simulink model "KTB1_EKF2b"  (R2022b)
settings: Solver=ode23tb  StartTime=0.0  StopTime=500  RelTol=1e-3
libraries: slpidlib x6
settings Model: Creator=s182032  LastModifiedBy=morebo
settings DataIOCC: ReturnWorkspaceOutputs=off
settings DebuggingCC: MaxConsecutiveZCsMsg=none  UnconnectedInputMsg=warning  UnconnectedOutputMsg=warning  UnconnectedLineMsg=warning  SFMachineParentedDataDiag=warning  ArithmeticOperatorsInVariantConditions=warning
settings ModelReferenceCC: EnableRefExpFcnMdlSchedulingChecks=on
settings SFSimCC: SimUseLocalCustomCode=off  CustomCodeUndefinedFunction=UseInterfaceOnly
settings RTWCC: RTWUseLocalCustomCode=off

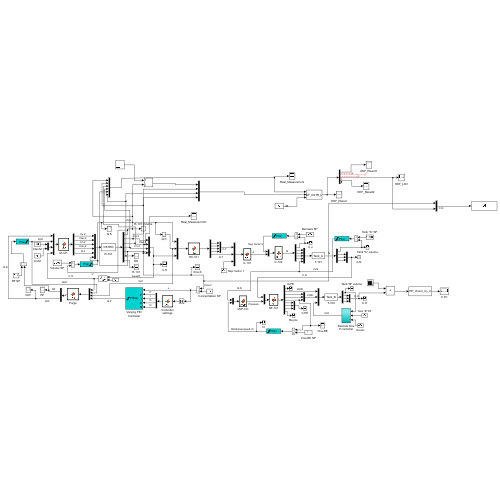
[thumbnail: Simulink's stored preview of the top-level diagram]
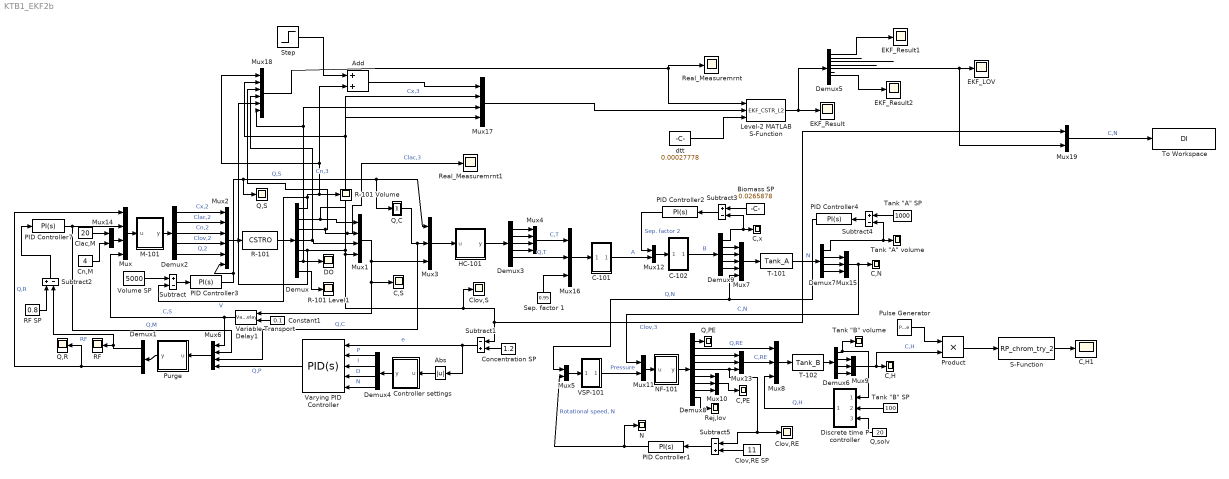
== system KTB1_EKF2b ==
  Abs : Abs  SaturateOnIntegerOverflow=off
  Add : Sum
  Biomass SP : Constant  Value=0.0265878
  C,H : Scope
  C,H1 : Scope
  C,N : Scope
  C,PE : Scope
  C,S : Scope
  C,x : Scope
  C-101 : MATLAB Function  TreatAsAtomicUnit=on
  C-102 : MATLAB Function  TreatAsAtomicUnit=on
  Clac,M : Constant  Value=20
  Clov,RE : Scope
  Clov,RE SP : Constant  Value=11
  Clov,S : Scope
  Cn,M : Constant  Value=4
  Concentration SP : Constant  Value=1.2
  Constant1 : Constant  Value=0.1
  Controller settings : MATLAB Function  TreatAsAtomicUnit=on
  DO : Scope
  Demux : Demux  Outputs=7
  Demux1 : Demux  Outputs=2
  Demux2 : Demux  Outputs=5
  Demux3 : Demux  Outputs=5
  Demux4 : Demux
  Demux5 : Demux  Outputs=8
  Demux6 : Demux
  Demux7 : Demux
  Demux8 : Demux  Outputs=9
  Demux9 : Demux  Outputs=5
  Discrete time P controller : Subsystem
  EKF_LOV : Scope
  EKF_Result : Scope
  EKF_Result1 : Scope
  EKF_Result2 : Scope
  HC-101 : MATLAB Function  TreatAsAtomicUnit=on
  Level-2 MATLAB S-Function : M-S-Function  FunctionName=EKF_CSTR_L2
  M-101 : MATLAB Function  TreatAsAtomicUnit=on
  Mux{,1,4,6,17} (5 alike) : Mux
  Mux{3,8..10,13,15..16} (7 alike) : Mux  Inputs=3
  Mux{5,11..12,14,19} (5 alike) : Mux  Inputs=2
  Mux18 : Mux  Inputs=6
  Mux2 : Mux  Inputs=6
  Mux7 : Mux  Inputs=5
  N : Scope
  NF-101 : MATLAB Function  TreatAsAtomicUnit=on
  PID Controller1 : slpidlib/PID Controller  Controller=PI  Form=Parallel  TimeDomain=Continuous-time  UseExternalTs=off  SampleTime=-1  IntegratorMethod=Forward Euler  FilterMethod=Forward Euler  ControllerParametersSource=internal  P=0.234567821807165  I=0.999999996666666*0.234567821807165  UseKiTs=off  D=0  N=100  UseFilter=on  TunerSelectOption=Transfer Function Based (PID Tuner App)  InitialConditionSource=internal  InitialConditionForIntegrator=3000  InitialConditionForFilter=0  DifferentiatorICPrevScaledInput=0  ExternalReset=none  TrackingMode=off  Kt=1  LimitOutput=on  SatLimitsSource=internal  UpperSaturationLimit=inf  LowerSaturationLimit=0  LinearizeAsGain=on  AntiWindupMode=clamping  Kb=1  LimitIntegrator=off  UpperIntegratorSaturationLimit=inf  LowerIntegratorSaturationLimit=-inf  POutMin=[]  POutMax=[]  IOutMin=[]  IOutMax=[]  DOutMin=[]  DOutMax=[]  NOutMin=[]  NOutMax=[]  SumOutMin=[]  SumOutMax=[]  SaturationOutMin=[]  SaturationOutMax=[]  PParamMin=[]  PParamMax=[]  IParamMin=[]  IParamMax=[]  DParamMin=[]  DParamMax=[]  NParamMin=[]  NParamMax=[]  KbParamMin=[]  KbParamMax=[]  KtParamMin=[]  KtParamMax=[]  KbOutMin=[]  KbOutMax=[]  KtOutMin=[]  KtOutMax=[]  IntegratorOutMin=[]  IntegratorOutMax=[]  FilterOutMin=[]  FilterOutMax=[]  SumI1OutMin=[]  SumI1OutMax=[]  SumI2OutMin=[]  SumI2OutMax=[]  SumI3OutMin=[]  SumI3OutMax=[]  SumI4OutMin=[]  SumI4OutMax=[]  SumDOutMin=[]  SumDOutMax=[]  DifferentiatorOutMin=[]  DifferentiatorOutMax=[]  FilterDiffOutCoefMin=[]  FilterDiffOutCoefMax=[]  ReciprocalOutMin=[]  ReciprocalOutMax=[]  SumDenOutMin=[]  SumDenOutMax=[]  SumNumOutMin=[]  SumNumOutMax=[]  DivideOutMin=[]  DivideOutMax=[]  UdiffTsProdOutMin=[]  UdiffTsProdOutMax=[]  NTsProdOutMin=[]  NTsProdOutMax=[]  UintegralTsProdOutMin=[]  UintegralTsProdOutMax=[]  UngainTsProdOutMin=[]  UngainTsProdOutMax=[]  ClampingZeroOutDataTypeStr=Inherit: Inherit via back propagation  ClampingZeroOutMin=[]  ClampingZeroOutMax=[]  FilterDenConstantOutDataTypeStr=Inherit: Inherit via back propagation  FilterDenConstantOutMin=[]  FilterDenConstantOutMax=[]  PCopyOutDataTypeStr=Inherit: Inherit via back propagation  PCopyOutMin=[]  PCopyOutMax=[]  NCopyOutDataTypeStr=Inherit: Inherit via back propagation  NCopyOutMin=[]  NCopyOutMax=[]  IntegratorContinuousStateAttributes=''  IntegratorStateMustResolveToSignalObject=off  IntegratorRTWStateStorageClass=Auto  FilterContinuousStateAttributes=''  FilterStateMustResolveToSignalObject=off  FilterRTWStateStorageClass=Auto  ParallelPVariant=InternalParameters  IdealPVariant=Disabled  IVariant=InternalParameters  DVariant=Disabled  IntegratorVariant=Continuous  SatVariant=Enabled  AWVariant=ContClampingParallel  PCopyVariant=Disabled  TRVariant=Disabled  FdbkBlocksVariant=Forward  IdealPFdbkVariant=Disabled  SatFdbkVariant=Disabled  DerivativeFilterVariant=Disabled  NVariant=Disabled  NCopyVariant=Disabled_SignalSpec  FilterICVariant=Disabled  IntegratorICVariant=InternalICs  ExternalResetVariant=Disabled  TRSumVariant=Passthrough  SumFdbkVariant=Disabled  SumVariant=Sum_PI  TsampFilterVariant=InternalTs  TsampNgainVariant=Passthrough  TsampIntegralVariant=Passthrough  ExternalSaturationOutDataTypeStr=Inherit: Same as second input
  PID Controller2 : slpidlib/PID Controller  Controller=PI  Form=Parallel  TimeDomain=Continuous-time  UseExternalTs=off  SampleTime=-1  IntegratorMethod=Forward Euler  FilterMethod=Forward Euler  ControllerParametersSource=internal  P=-0.000476190628986061  I=9.99999996666667*(-0.000476190628986061)  UseKiTs=off  D=0  N=100  UseFilter=on  TunerSelectOption=Transfer Function Based (PID Tuner App)  InitialConditionSource=internal  InitialConditionForIntegrator=0.95  InitialConditionForFilter=0  DifferentiatorICPrevScaledInput=0  ExternalReset=none  TrackingMode=off  Kt=1  LimitOutput=on  SatLimitsSource=internal  UpperSaturationLimit=0.98  LowerSaturationLimit=0  LinearizeAsGain=on  AntiWindupMode=clamping  Kb=1  LimitIntegrator=off  UpperIntegratorSaturationLimit=inf  LowerIntegratorSaturationLimit=-inf  POutMin=[]  POutMax=[]  IOutMin=[]  IOutMax=[]  DOutMin=[]  DOutMax=[]  NOutMin=[]  NOutMax=[]  SumOutMin=[]  SumOutMax=[]  SaturationOutMin=[]  SaturationOutMax=[]  PParamMin=[]  PParamMax=[]  IParamMin=[]  IParamMax=[]  DParamMin=[]  DParamMax=[]  NParamMin=[]  NParamMax=[]  KbParamMin=[]  KbParamMax=[]  KtParamMin=[]  KtParamMax=[]  KbOutMin=[]  KbOutMax=[]  KtOutMin=[]  KtOutMax=[]  IntegratorOutMin=[]  IntegratorOutMax=[]  FilterOutMin=[]  FilterOutMax=[]  SumI1OutMin=[]  SumI1OutMax=[]  SumI2OutMin=[]  SumI2OutMax=[]  SumI3OutMin=[]  SumI3OutMax=[]  SumI4OutMin=[]  SumI4OutMax=[]  SumDOutMin=[]  SumDOutMax=[]  DifferentiatorOutMin=[]  DifferentiatorOutMax=[]  FilterDiffOutCoefMin=[]  FilterDiffOutCoefMax=[]  ReciprocalOutMin=[]  ReciprocalOutMax=[]  SumDenOutMin=[]  SumDenOutMax=[]  SumNumOutMin=[]  SumNumOutMax=[]  DivideOutMin=[]  DivideOutMax=[]  UdiffTsProdOutMin=[]  UdiffTsProdOutMax=[]  NTsProdOutMin=[]  NTsProdOutMax=[]  UintegralTsProdOutMin=[]  UintegralTsProdOutMax=[]  UngainTsProdOutMin=[]  UngainTsProdOutMax=[]  ClampingZeroOutDataTypeStr=Inherit: Inherit via back propagation  ClampingZeroOutMin=[]  ClampingZeroOutMax=[]  FilterDenConstantOutDataTypeStr=Inherit: Inherit via back propagation  FilterDenConstantOutMin=[]  FilterDenConstantOutMax=[]  PCopyOutDataTypeStr=Inherit: Inherit via back propagation  PCopyOutMin=[]  PCopyOutMax=[]  NCopyOutDataTypeStr=Inherit: Inherit via back propagation  NCopyOutMin=[]  NCopyOutMax=[]  IntegratorContinuousStateAttributes=''  IntegratorStateMustResolveToSignalObject=off  IntegratorRTWStateStorageClass=Auto  FilterContinuousStateAttributes=''  FilterStateMustResolveToSignalObject=off  FilterRTWStateStorageClass=Auto  ParallelPVariant=InternalParameters  IdealPVariant=Disabled  IVariant=InternalParameters  DVariant=Disabled  IntegratorVariant=Continuous  SatVariant=Enabled  AWVariant=ContClampingParallel  PCopyVariant=Disabled  TRVariant=Disabled  FdbkBlocksVariant=Forward  IdealPFdbkVariant=Disabled  SatFdbkVariant=Disabled  DerivativeFilterVariant=Disabled  NVariant=Disabled  NCopyVariant=Disabled_SignalSpec  FilterICVariant=Disabled  IntegratorICVariant=InternalICs  ExternalResetVariant=Disabled  TRSumVariant=Passthrough  SumFdbkVariant=Disabled  SumVariant=Sum_PI  TsampFilterVariant=InternalTs  TsampNgainVariant=Passthrough  TsampIntegralVariant=Passthrough  ExternalSaturationOutDataTypeStr=Inherit: Same as second input
  PID Controller3 : slpidlib/PID Controller  Controller=PI  Form=Parallel  TimeDomain=Continuous-time  UseExternalTs=off  SampleTime=-1  IntegratorMethod=Forward Euler  FilterMethod=Forward Euler  ControllerParametersSource=internal  P=-1/0.4/0.2  I=-1/0.4/0.2/4/0.2  UseKiTs=off  D=0  N=100  UseFilter=on  TunerSelectOption=Transfer Function Based (PID Tuner App)  InitialConditionSource=internal  InitialConditionForIntegrator=64.0830509473650  InitialConditionForFilter=0  DifferentiatorICPrevScaledInput=0  ExternalReset=none  TrackingMode=off  Kt=1  LimitOutput=on  SatLimitsSource=internal  UpperSaturationLimit=inf  LowerSaturationLimit=0  LinearizeAsGain=on  AntiWindupMode=clamping  Kb=1  LimitIntegrator=off  UpperIntegratorSaturationLimit=inf  LowerIntegratorSaturationLimit=-inf  POutMin=[]  POutMax=[]  IOutMin=[]  IOutMax=[]  DOutMin=[]  DOutMax=[]  NOutMin=[]  NOutMax=[]  SumOutMin=[]  SumOutMax=[]  SaturationOutMin=[]  SaturationOutMax=[]  PParamMin=[]  PParamMax=[]  IParamMin=[]  IParamMax=[]  DParamMin=[]  DParamMax=[]  NParamMin=[]  NParamMax=[]  KbParamMin=[]  KbParamMax=[]  KtParamMin=[]  KtParamMax=[]  KbOutMin=[]  KbOutMax=[]  KtOutMin=[]  KtOutMax=[]  IntegratorOutMin=[]  IntegratorOutMax=[]  FilterOutMin=[]  FilterOutMax=[]  SumI1OutMin=[]  SumI1OutMax=[]  SumI2OutMin=[]  SumI2OutMax=[]  SumI3OutMin=[]  SumI3OutMax=[]  SumI4OutMin=[]  SumI4OutMax=[]  SumDOutMin=[]  SumDOutMax=[]  DifferentiatorOutMin=[]  DifferentiatorOutMax=[]  FilterDiffOutCoefMin=[]  FilterDiffOutCoefMax=[]  ReciprocalOutMin=[]  ReciprocalOutMax=[]  SumDenOutMin=[]  SumDenOutMax=[]  SumNumOutMin=[]  SumNumOutMax=[]  DivideOutMin=[]  DivideOutMax=[]  UdiffTsProdOutMin=[]  UdiffTsProdOutMax=[]  NTsProdOutMin=[]  NTsProdOutMax=[]  UintegralTsProdOutMin=[]  UintegralTsProdOutMax=[]  UngainTsProdOutMin=[]  UngainTsProdOutMax=[]  ClampingZeroOutDataTypeStr=Inherit: Inherit via back propagation  ClampingZeroOutMin=[]  ClampingZeroOutMax=[]  FilterDenConstantOutDataTypeStr=Inherit: Inherit via back propagation  FilterDenConstantOutMin=[]  FilterDenConstantOutMax=[]  PCopyOutDataTypeStr=Inherit: Inherit via back propagation  PCopyOutMin=[]  PCopyOutMax=[]  NCopyOutDataTypeStr=Inherit: Inherit via back propagation  NCopyOutMin=[]  NCopyOutMax=[]  IntegratorContinuousStateAttributes=''  IntegratorStateMustResolveToSignalObject=off  IntegratorRTWStateStorageClass=Auto  FilterContinuousStateAttributes=''  FilterStateMustResolveToSignalObject=off  FilterRTWStateStorageClass=Auto  ParallelPVariant=InternalParameters  IdealPVariant=Disabled  IVariant=InternalParameters  DVariant=Disabled  IntegratorVariant=Continuous  SatVariant=Enabled  AWVariant=ContClampingParallel  PCopyVariant=Disabled  TRVariant=Disabled  FdbkBlocksVariant=Forward  IdealPFdbkVariant=Disabled  SatFdbkVariant=Disabled  DerivativeFilterVariant=Disabled  NVariant=Disabled  NCopyVariant=Disabled_SignalSpec  FilterICVariant=Disabled  IntegratorICVariant=InternalICs  ExternalResetVariant=Disabled  TRSumVariant=Passthrough  SumFdbkVariant=Disabled  SumVariant=Sum_PI  TsampFilterVariant=InternalTs  TsampNgainVariant=Passthrough  TsampIntegralVariant=Passthrough  ExternalSaturationOutDataTypeStr=Inherit: Same as second input
  PID Controller4 : slpidlib/PID Controller  Controller=PI  Form=Parallel  TimeDomain=Continuous-time  UseExternalTs=off  SampleTime=-1  IntegratorMethod=Forward Euler  FilterMethod=Forward Euler  ControllerParametersSource=internal  P=-1/140  I=-1/4/140/140  UseKiTs=off  D=0  N=100  UseFilter=on  TunerSelectOption=Transfer Function Based (PID Tuner App)  InitialConditionSource=internal  InitialConditionForIntegrator=25.6332203789471  InitialConditionForFilter=0  DifferentiatorICPrevScaledInput=0  ExternalReset=none  TrackingMode=off  Kt=1  LimitOutput=on  SatLimitsSource=internal  UpperSaturationLimit=inf  LowerSaturationLimit=0  LinearizeAsGain=on  AntiWindupMode=clamping  Kb=1  LimitIntegrator=off  UpperIntegratorSaturationLimit=inf  LowerIntegratorSaturationLimit=-inf  POutMin=[]  POutMax=[]  IOutMin=[]  IOutMax=[]  DOutMin=[]  DOutMax=[]  NOutMin=[]  NOutMax=[]  SumOutMin=[]  SumOutMax=[]  SaturationOutMin=[]  SaturationOutMax=[]  PParamMin=[]  PParamMax=[]  IParamMin=[]  IParamMax=[]  DParamMin=[]  DParamMax=[]  NParamMin=[]  NParamMax=[]  KbParamMin=[]  KbParamMax=[]  KtParamMin=[]  KtParamMax=[]  KbOutMin=[]  KbOutMax=[]  KtOutMin=[]  KtOutMax=[]  IntegratorOutMin=[]  IntegratorOutMax=[]  FilterOutMin=[]  FilterOutMax=[]  SumI1OutMin=[]  SumI1OutMax=[]  SumI2OutMin=[]  SumI2OutMax=[]  SumI3OutMin=[]  SumI3OutMax=[]  SumI4OutMin=[]  SumI4OutMax=[]  SumDOutMin=[]  SumDOutMax=[]  DifferentiatorOutMin=[]  DifferentiatorOutMax=[]  FilterDiffOutCoefMin=[]  FilterDiffOutCoefMax=[]  ReciprocalOutMin=[]  ReciprocalOutMax=[]  SumDenOutMin=[]  SumDenOutMax=[]  SumNumOutMin=[]  SumNumOutMax=[]  DivideOutMin=[]  DivideOutMax=[]  UdiffTsProdOutMin=[]  UdiffTsProdOutMax=[]  NTsProdOutMin=[]  NTsProdOutMax=[]  UintegralTsProdOutMin=[]  UintegralTsProdOutMax=[]  UngainTsProdOutMin=[]  UngainTsProdOutMax=[]  ClampingZeroOutDataTypeStr=Inherit: Inherit via back propagation  ClampingZeroOutMin=[]  ClampingZeroOutMax=[]  FilterDenConstantOutDataTypeStr=Inherit: Inherit via back propagation  FilterDenConstantOutMin=[]  FilterDenConstantOutMax=[]  PCopyOutDataTypeStr=Inherit: Inherit via back propagation  PCopyOutMin=[]  PCopyOutMax=[]  NCopyOutDataTypeStr=Inherit: Inherit via back propagation  NCopyOutMin=[]  NCopyOutMax=[]  IntegratorContinuousStateAttributes=''  IntegratorStateMustResolveToSignalObject=off  IntegratorRTWStateStorageClass=Auto  FilterContinuousStateAttributes=''  FilterStateMustResolveToSignalObject=off  FilterRTWStateStorageClass=Auto  ParallelPVariant=InternalParameters  IdealPVariant=Disabled  IVariant=InternalParameters  DVariant=Disabled  IntegratorVariant=Continuous  SatVariant=Enabled  AWVariant=ContClampingParallel  PCopyVariant=Disabled  TRVariant=Disabled  FdbkBlocksVariant=Forward  IdealPFdbkVariant=Disabled  SatFdbkVariant=Disabled  DerivativeFilterVariant=Disabled  NVariant=Disabled  NCopyVariant=Disabled_SignalSpec  FilterICVariant=Disabled  IntegratorICVariant=InternalICs  ExternalResetVariant=Disabled  TRSumVariant=Passthrough  SumFdbkVariant=Disabled  SumVariant=Sum_PI  TsampFilterVariant=InternalTs  TsampNgainVariant=Passthrough  TsampIntegralVariant=Passthrough  ExternalSaturationOutDataTypeStr=Inherit: Same as second input
  PID Controller7 : slpidlib/PID Controller  Controller=PI  Form=Parallel  TimeDomain=Continuous-time  UseExternalTs=off  SampleTime=-1  IntegratorMethod=Forward Euler  FilterMethod=Forward Euler  ControllerParametersSource=internal  P=4.68116891262785/100  I=30.3539293345611/100  UseKiTs=off  D=0  N=100  UseFilter=on  TunerSelectOption=Transfer Function Based (PID Tuner App)  InitialConditionSource=internal  InitialConditionForIntegrator=35.6016949707568  InitialConditionForFilter=0  DifferentiatorICPrevScaledInput=0  ExternalReset=none  TrackingMode=off  Kt=1  LimitOutput=on  SatLimitsSource=internal  UpperSaturationLimit=inf  LowerSaturationLimit=0  LinearizeAsGain=on  AntiWindupMode=clamping  Kb=1  LimitIntegrator=off  UpperIntegratorSaturationLimit=inf  LowerIntegratorSaturationLimit=-inf  POutMin=[]  POutMax=[]  IOutMin=[]  IOutMax=[]  DOutMin=[]  DOutMax=[]  NOutMin=[]  NOutMax=[]  SumOutMin=[]  SumOutMax=[]  SaturationOutMin=[]  SaturationOutMax=[]  PParamMin=[]  PParamMax=[]  IParamMin=[]  IParamMax=[]  DParamMin=[]  DParamMax=[]  NParamMin=[]  NParamMax=[]  KbParamMin=[]  KbParamMax=[]  KtParamMin=[]  KtParamMax=[]  KbOutMin=[]  KbOutMax=[]  KtOutMin=[]  KtOutMax=[]  IntegratorOutMin=[]  IntegratorOutMax=[]  FilterOutMin=[]  FilterOutMax=[]  SumI1OutMin=[]  SumI1OutMax=[]  SumI2OutMin=[]  SumI2OutMax=[]  SumI3OutMin=[]  SumI3OutMax=[]  SumI4OutMin=[]  SumI4OutMax=[]  SumDOutMin=[]  SumDOutMax=[]  DifferentiatorOutMin=[]  DifferentiatorOutMax=[]  FilterDiffOutCoefMin=[]  FilterDiffOutCoefMax=[]  ReciprocalOutMin=[]  ReciprocalOutMax=[]  SumDenOutMin=[]  SumDenOutMax=[]  SumNumOutMin=[]  SumNumOutMax=[]  DivideOutMin=[]  DivideOutMax=[]  UdiffTsProdOutMin=[]  UdiffTsProdOutMax=[]  NTsProdOutMin=[]  NTsProdOutMax=[]  UintegralTsProdOutMin=[]  UintegralTsProdOutMax=[]  UngainTsProdOutMin=[]  UngainTsProdOutMax=[]  ClampingZeroOutDataTypeStr=Inherit: Inherit via back propagation  ClampingZeroOutMin=[]  ClampingZeroOutMax=[]  FilterDenConstantOutDataTypeStr=Inherit: Inherit via back propagation  FilterDenConstantOutMin=[]  FilterDenConstantOutMax=[]  PCopyOutDataTypeStr=Inherit: Inherit via back propagation  PCopyOutMin=[]  PCopyOutMax=[]  NCopyOutDataTypeStr=Inherit: Inherit via back propagation  NCopyOutMin=[]  NCopyOutMax=[]  IntegratorContinuousStateAttributes=''  IntegratorStateMustResolveToSignalObject=off  IntegratorRTWStateStorageClass=Auto  FilterContinuousStateAttributes=''  FilterStateMustResolveToSignalObject=off  FilterRTWStateStorageClass=Auto  ParallelPVariant=InternalParameters  IdealPVariant=Disabled  IVariant=InternalParameters  DVariant=Disabled  IntegratorVariant=Continuous  SatVariant=Enabled  AWVariant=ContClampingParallel  PCopyVariant=Disabled  TRVariant=Disabled  FdbkBlocksVariant=Forward  IdealPFdbkVariant=Disabled  SatFdbkVariant=Disabled  DerivativeFilterVariant=Disabled  NVariant=Disabled  NCopyVariant=Disabled_SignalSpec  FilterICVariant=Disabled  IntegratorICVariant=InternalICs  ExternalResetVariant=Disabled  TRSumVariant=Passthrough  SumFdbkVariant=Disabled  SumVariant=Sum_PI  TsampFilterVariant=InternalTs  TsampNgainVariant=Passthrough  TsampIntegralVariant=Passthrough  ExternalSaturationOutDataTypeStr=Inherit: Same as second input
  Product : Product
  Pulse Generator : DiscretePulseGenerator  PulseType=Time based  Period=12  PulseWidth=12.833
  Purge : MATLAB Function  TreatAsAtomicUnit=on
  Q,C : Subsystem
  Q,PE : Scope
  Q,R : Scope
  Q,S : Scope
  Q,solv : Constant  Value=20
  R-101 : S-Function  FunctionName=CSTRO  SFunctionDeploymentMode=off  EnableBusSupport=off
  R-101 Level1 : Scope
  R-101 Volume : Scope
  RF : Scope
  RF SP : Constant  Value=0.8
  Real_Measuremrnt : Scope
  Real_Measuremrnt1 : Scope
  Rej,lov : Scope
  S-Function : S-Function  FunctionName=RP_chrom_try_2  Parameters=50  SFunctionDeploymentMode=off  EnableBusSupport=off
  Sep. factor 1 : Constant  Value=0.95
  Step : Step  Time=50  After=50  SampleTime=0
  Subtract{,2..4} (4 alike) : Sum  Inputs=+-
  Subtract1 : Sum  Inputs=-+
  Subtract5 : Sum  Inputs=-+
  T-101 : S-Function  FunctionName=Tank_A  SFunctionDeploymentMode=off  EnableBusSupport=off
  T-102 : S-Function  FunctionName=Tank_B  SFunctionDeploymentMode=off  EnableBusSupport=off
  "Tank \"A\" SP" : Constant  Value=1000
  "Tank \"A\" volume" : Scope
  "Tank \"B\" SP" : Constant  Value=100
  "Tank \"B\" volume" : Scope
  To Workspace : ToWorkspace  VariableName=DI  SaveFormat=Timeseries  SampleTime=-1
  VSP-101 : MATLAB Function  TreatAsAtomicUnit=on
  Variable Transport Delay1 : VariableTransportDelay  VariableDelayType=Variable transport delay  MaximumDelay=10  InitialOutput=[106.351163614666 14.8096563646109 2.51553709810012 1.20000000000003]  MaximumPoints=80000
  Varying PID Controller : slpidlib/PID Controller  Controller=PID  Form=Parallel  TimeDomain=Continuous-time  UseExternalTs=off  SampleTime=-1  IntegratorMethod=Forward Euler  FilterMethod=Forward Euler  ControllerParametersSource=external  P=1  I=1  UseKiTs=off  D=0  N=100  UseFilter=on  TunerSelectOption=Transfer Function Based (PID Tuner App)  InitialConditionSource=internal  InitialConditionForIntegrator=9.96847459181301  InitialConditionForFilter=0  DifferentiatorICPrevScaledInput=0  ExternalReset=none  TrackingMode=off  Kt=1  LimitOutput=on  SatLimitsSource=internal  UpperSaturationLimit=inf  LowerSaturationLimit=0  LinearizeAsGain=on  AntiWindupMode=none  Kb=1  LimitIntegrator=off  UpperIntegratorSaturationLimit=inf  LowerIntegratorSaturationLimit=-inf  POutMin=[]  POutMax=[]  IOutMin=[]  IOutMax=[]  DOutMin=[]  DOutMax=[]  NOutMin=[]  NOutMax=[]  SumOutMin=[]  SumOutMax=[]  SaturationOutMin=[]  SaturationOutMax=[]  PParamMin=[]  PParamMax=[]  IParamMin=[]  IParamMax=[]  DParamMin=[]  DParamMax=[]  NParamMin=[]  NParamMax=[]  KbParamMin=[]  KbParamMax=[]  KtParamMin=[]  KtParamMax=[]  KbOutMin=[]  KbOutMax=[]  KtOutMin=[]  KtOutMax=[]  IntegratorOutMin=[]  IntegratorOutMax=[]  FilterOutMin=[]  FilterOutMax=[]  SumI1OutMin=[]  SumI1OutMax=[]  SumI2OutMin=[]  SumI2OutMax=[]  SumI3OutMin=[]  SumI3OutMax=[]  SumI4OutMin=[]  SumI4OutMax=[]  SumDOutMin=[]  SumDOutMax=[]  DifferentiatorOutMin=[]  DifferentiatorOutMax=[]  FilterDiffOutCoefMin=[]  FilterDiffOutCoefMax=[]  ReciprocalOutMin=[]  ReciprocalOutMax=[]  SumDenOutMin=[]  SumDenOutMax=[]  SumNumOutMin=[]  SumNumOutMax=[]  DivideOutMin=[]  DivideOutMax=[]  UdiffTsProdOutMin=[]  UdiffTsProdOutMax=[]  NTsProdOutMin=[]  NTsProdOutMax=[]  UintegralTsProdOutMin=[]  UintegralTsProdOutMax=[]  UngainTsProdOutMin=[]  UngainTsProdOutMax=[]  ClampingZeroOutDataTypeStr=Inherit: Inherit via back propagation  ClampingZeroOutMin=[]  ClampingZeroOutMax=[]  FilterDenConstantOutDataTypeStr=Inherit: Inherit via back propagation  FilterDenConstantOutMin=[]  FilterDenConstantOutMax=[]  PCopyOutDataTypeStr=Inherit: Inherit via back propagation  PCopyOutMin=[]  PCopyOutMax=[]  NCopyOutDataTypeStr=Inherit: Inherit via back propagation  NCopyOutMin=[]  NCopyOutMax=[]  IntegratorContinuousStateAttributes=''  IntegratorStateMustResolveToSignalObject=off  IntegratorRTWStateStorageClass=Auto  FilterContinuousStateAttributes=''  FilterStateMustResolveToSignalObject=off  FilterRTWStateStorageClass=Auto  ParallelPVariant=ExternalParameters  IdealPVariant=Disabled  IVariant=ExternalParameters  DVariant=ExternalParameters  IntegratorVariant=Continuous  SatVariant=Enabled  AWVariant=Passthrough  PCopyVariant=Disabled  TRVariant=Disabled  FdbkBlocksVariant=Forward  IdealPFdbkVariant=Disabled  SatFdbkVariant=Disabled  DerivativeFilterVariant=ContFilter  NVariant=ExternalParameters  NCopyVariant=Disabled  FilterICVariant=InternalICsFilter  IntegratorICVariant=InternalICs  ExternalResetVariant=Disabled  TRSumVariant=Passthrough  SumFdbkVariant=Disabled  SumVariant=Sum_PID  TsampFilterVariant=InternalTs  TsampNgainVariant=Passthrough  TsampIntegralVariant=Passthrough  ExternalSaturationOutDataTypeStr=Inherit: Same as second input
  Volume SP : Constant  Value=5000
  dtt : Constant  Value=0.00027778
  wires:
  Concentration SP/1 -> Subtract1/2
  Demux4/1 -> Varying PID Controller/2  "P"
  Subtract1/1 -> Abs/1, Varying PID Controller/1  "e"
  Demux4/2 -> Varying PID Controller/3  "I"
  PID Controller7/1 -> Mux6/2, Mux/2  "Q,M"
  Varying PID Controller/1 -> Mux6/4  "Q,P"
  Demux2/5 -> Mux2/5  "Q,2"
  Mux6/1 -> Purge/1(u)
  Demux2/4 -> Mux2/4  "Clov,2"
  Demux3/1 -> Mux4/1
  Purge/1(y) -> Demux1/1
  Demux2/3 -> Mux2/3  "Cn,2"
  Demux3/2 -> Mux4/2
  Demux3/3 -> Mux4/3
  HC-101/1(y) -> Demux3/1
  Mux3/1 -> HC-101/1(u)
  Demux2/2 -> Mux2/2  "Clac,2"
  PID Controller3/1 -> Mux2/6, Q,C/1(Qs), Mux3/1, Q,S/1  "Q,S"
  Demux/1 -> Add/2, Mux18/1, R-101 Volume/1, Subtract/2  "V"
  Demux/2 -> Mux17/2, Mux18/2, Mux1/1  "Cx,3"
  Demux/3 -> Mux18/3, Real_Measuremrnt1/1, Mux1/2  "Clac,3"
  Mux/1 -> M-101/1(u)
  Mux2/1 -> R-101/1
  Demux2/1 -> Mux2/1  "Cx,2"
  Variable Transport Delay1/1 -> Mux/4, Mux6/1  "C,S"
  R-101/1 -> Demux/1
  Mux1/1 -> C,S/1, Variable Transport Delay1/1, Mux3/3
  Constant1/1 -> Variable Transport Delay1/2
  M-101/1(y) -> Demux2/1
  Demux/4 -> Mux18/4, Mux1/3  "Cn,3"
  Demux/5 -> Mux19/1, Subtract1/1, Clov,S/1, Mux1/4, Mux17/4, Mux18/5  "Clov,3"
  Subtract/1 -> PID Controller3/1
  Demux3/4 -> Mux4/4
  Demux/6 -> DO/1, Mux17/3, Mux18/6
  Mux14/1 -> Mux/3
  Demux1/2 -> Mux/1, Q,R/1  "Q,R"
  Volume SP/1 -> Subtract/1
  Demux1/1 -> Subtract2/2, RF/1  "RF"
  Clac,M/1 -> Mux14/1
  Abs/1 -> Controller settings/1(u)
  Controller settings/1(y) -> Demux4/1
  Demux4/3 -> Varying PID Controller/4  "D"
  Demux4/4 -> Varying PID Controller/5  "N"
  RF SP/1 -> Subtract2/1
  Subtract2/1 -> PID Controller7/1
  Q,C/1(Qc) -> Mux6/3, Mux3/2  "Q,C"
  Demux6/1 -> Discrete time P controller/1(In1), "Tank \"B\" volume"/1
  Discrete time P controller/1(Q,H) -> Mux8/3  "Q,H"
  Q,solv/1 -> Discrete time P controller/3(In3)
  "Tank \"B\" SP"/1 -> Discrete time P controller/2(In2)
  Demux9/4 -> Mux7/3
  Clov,RE SP/1 -> Subtract5/2
  Subtract3/1 -> PID Controller2/1
  C-102/1(y) -> Demux9/1  "B"
  Demux8/9 -> Rej,lov/1
  PID Controller1/1 -> Mux5/2, N/1  "Rotational speed, N"
  Demux9/1 -> Subtract3/2, C,x/1
  Demux7/3 -> Mux15/2
  Demux8/8 -> Mux10/3
  Demux9/2 -> Mux7/1
  Mux5/1 -> VSP-101/1(u)
  VSP-101/1(y) -> Mux11/2  "Pressure"
  Demux6/2 -> Mux9/1
  T-102/1 -> Demux6/1
  Demux9/5 -> Mux7/4
  Demux8/2 -> Mux8/1  "Q,RE"
  Demux6/3 -> Mux9/2
  Mux15/1 -> Mux11/1, C,N/1  "C,N"
  Mux7/1 -> T-101/1
  Demux9/3 -> Mux7/2
  Demux8/3 -> Mux13/1
  Demux8/5 -> Clov,RE/1, Subtract5/1, Mux13/3
  Mux8/1 -> T-102/1
  Mux10/1 -> C,PE/1
  Demux8/4 -> Mux13/2
  Subtract4/1 -> PID Controller4/1
  PID Controller4/1 -> Mux5/1, Mux7/5  "Q,N"
  Subtract5/1 -> PID Controller1/1
  Demux8/7 -> Mux10/2
  Demux6/4 -> Mux9/3
  Demux7/1 -> "Tank \"A\" volume"/1, Subtract4/2
  Mux16/1 -> C-101/1(u)
  Sep. factor 1/1 -> Mux16/3
  Mux11/1 -> NF-101/1(u)
  NF-101/1(y) -> Demux8/1
  "Tank \"A\" SP"/1 -> Subtract4/1
  Mux9/1 -> Product/2, C,H/1  "C,H"
  T-101/1 -> Demux7/1  "N"
  Mux13/1 -> Mux8/2  "C,RE"
  Mux12/1 -> C-102/1(u)
  Biomass SP/1 -> Subtract3/1
  Demux8/6 -> Mux10/1
  Demux7/4 -> Mux15/3
  Demux8/1 -> Q,PE/1
  C-101/1(y) -> Mux12/2  "A"
  Demux7/2 -> Mux15/1
  PID Controller2/1 -> Mux12/1  "Sep. factor 2"
  Mux4/1 -> Mux16/1  "C,T"
  Demux3/5 -> Mux16/2  "Q,T"
  S-Function/1 -> C,H1/1
  Pulse Generator/1 -> Product/1
  Product/1 -> S-Function/1
  Demux/7 -> R-101 Level1/1
  Mux17/1 -> Level-2 MATLAB S-Function/2
  Mux18/1 -> Level-2 MATLAB S-Function/1, Real_Measuremrnt/1
  dtt/1 -> Level-2 MATLAB S-Function/3
  Level-2 MATLAB S-Function/1 -> Demux5/1, EKF_Result/1
  Demux5/1 -> EKF_Result1/1
  Demux5/4 -> ?
  Demux5/6 -> ?
  Demux5/2 -> ?
  Demux5/3 -> ?
  Demux5/5 -> Mux19/2, EKF_LOV/1
  Cn,M/1 -> Mux14/2
  Demux5/7 -> EKF_Result2/1
  Step/1 -> Add/1
  Add/1 -> Mux17/1
  Mux19/1 -> To Workspace/1  "C,N"

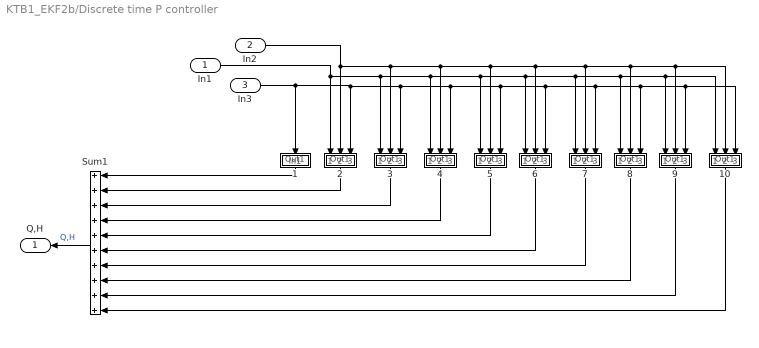
== system KTB1_EKF2b/Discrete time P controller ==
  In1 : Inport
  In2 : Inport  Port=2
  In3 : Inport  Port=3
  1 : Subsystem
  10 : Subsystem
  2 : Subsystem
  3 : Subsystem
  4 : Subsystem
  5 : Subsystem
  6 : Subsystem
  7 : Subsystem
  8 : Subsystem
  9 : Subsystem
  Sum1 : Sum  Inputs=++++++++++
  Q,H : Outport  VectorParamsAs1DForOutWhenUnconnected=off
  wires:
  In3/1 -> 3/3(In3), 4/3(In3), 6/3(In3), 7/3(In3), 8/3(In3), 10/3(In3), 9/3(In3), 5/3(In3), 2/3(In3), 1/1(In1)
  In2/1 -> 2/2(In2), 3/2(In2), 4/2(In2), 5/2(In2), 6/2(In2), 8/2(In2), 10/2(In2), 9/2(In2), 7/2(In2)
  7/1(Out1) -> Sum1/7
  3/1(Out1) -> Sum1/3
  4/1(Out1) -> Sum1/4
  2/1(Out1) -> Sum1/2
  6/1(Out1) -> Sum1/6
  8/1(Out1) -> Sum1/8
  10/1(Out1) -> Sum1/10
  9/1(Out1) -> Sum1/9
  5/1(Out1) -> Sum1/5
  Sum1/1 -> Q,H/1  "Q,H"
  1/1(Out1) -> Sum1/1
  In1/1 -> 4/1(In1), 5/1(In1), 6/1(In1), 7/1(In1), 8/1(In1), 10/1(In1), 9/1(In1), 3/1(In1), 2/1(In1)

== system KTB1_EKF2b/Q,C ==
  Qs : Inport
  Product1 : Product
  Q,C/Q,S : Constant  Value=0.6
  Qc : Outport  VectorParamsAs1DForOutWhenUnconnected=off
  wires:
  Product1/1 -> Qc/1  "Qc"
  Q,C/Q,S/1 -> Product1/1
  Qs/1 -> Product1/2

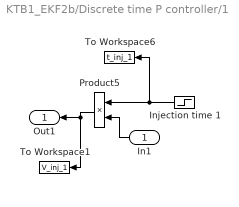
== system KTB1_EKF2b/Discrete time P controller/1 ==
  In1 : Inport
  Injection time 1 : Step  Time=(5.1313509526065/20)*6  Before=1  After=0  SampleTime=0
  Product5 : Product
  To Workspace1 : ToWorkspace  VariableName=V_inj_1  SaveFormat=Timeseries  SampleTime=-1
  To Workspace6 : ToWorkspace  VariableName=t_inj_1  SaveFormat=Timeseries  SampleTime=-1
  Out1 : Outport  VectorParamsAs1DForOutWhenUnconnected=off
  wires:
  Product5/1 -> To Workspace1/1, Out1/1
  Injection time 1/1 -> Product5/1, To Workspace6/1
  In1/1 -> Product5/2

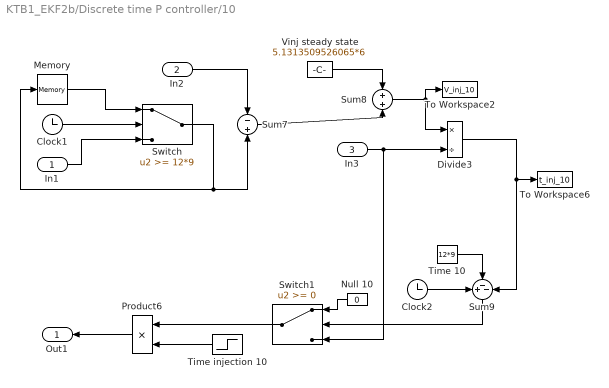
== system KTB1_EKF2b/Discrete time P controller/10 ==
  In1 : Inport
  In2 : Inport  Port=2
  In3 : Inport  Port=3
  Clock1 : Clock
  Clock2 : Clock
  Divide3 : Product  Inputs=*/
  Memory : Memory
  Null 10 : Constant  Value=0
  Product6 : Product
  Sum7 : Sum  Inputs=-+
  Sum8 : Sum
  Sum9 : Sum  Inputs=+--
  Switch : Switch  Threshold=12*9  SaturateOnIntegerOverflow=off  InputSameDT=off
  Switch1 : Switch  SaturateOnIntegerOverflow=off  InputSameDT=off
  Time 10 : Constant  Value=12*9
  Time injection 10 : Step  Time=12*9  SampleTime=0
  To Workspace2 : ToWorkspace  VariableName=V_inj_10  SaveFormat=Timeseries  SampleTime=-1
  To Workspace6 : ToWorkspace  VariableName=t_inj_10  SaveFormat=Timeseries  SampleTime=-1
  Vinj steady state : Constant  Value=5.1313509526065*6
  Out1 : Outport  VectorParamsAs1DForOutWhenUnconnected=off
  wires:
  In1/1 -> Switch/3
  Time injection 10/1 -> Product6/2
  Switch/1 -> Memory/1, Sum7/2
  Time 10/1 -> Sum9/2
  Switch1/1 -> Product6/1
  Clock1/1 -> Switch/2
  Memory/1 -> Switch/1
  Null 10/1 -> Switch1/1
  Divide3/1 -> Sum9/3, To Workspace6/1
  Clock2/1 -> Sum9/1
  In2/1 -> Sum7/1
  Vinj steady state/1 -> Sum8/1
  In3/1 -> Switch1/3, Divide3/2
  Sum9/1 -> Switch1/2
  Sum7/1 -> Sum8/2
  Product6/1 -> Out1/1
  Sum8/1 -> Divide3/1, To Workspace2/1

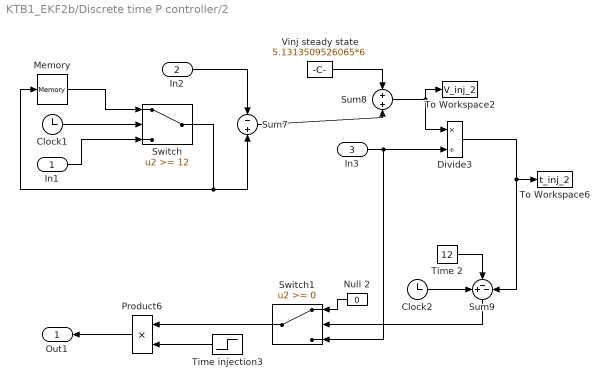
== system KTB1_EKF2b/Discrete time P controller/2 ==
  In1 : Inport
  In2 : Inport  Port=2
  In3 : Inport  Port=3
  Clock1 : Clock
  Clock2 : Clock
  Divide3 : Product  Inputs=*/
  Memory : Memory
  Null 2 : Constant  Value=0
  Product6 : Product
  Sum7 : Sum  Inputs=-+
  Sum8 : Sum
  Sum9 : Sum  Inputs=+--
  Switch : Switch  Threshold=12  SaturateOnIntegerOverflow=off  InputSameDT=off
  Switch1 : Switch  SaturateOnIntegerOverflow=off  InputSameDT=off
  Time 2 : Constant  Value=12
  Time injection3 : Step  Time=12  SampleTime=0
  To Workspace2 : ToWorkspace  VariableName=V_inj_2  SaveFormat=Timeseries  SampleTime=-1
  To Workspace6 : ToWorkspace  VariableName=t_inj_2  SaveFormat=Timeseries  SampleTime=-1
  Vinj steady state : Constant  Value=5.1313509526065*6
  Out1 : Outport  VectorParamsAs1DForOutWhenUnconnected=off
  wires:
  In1/1 -> Switch/3
  Time injection3/1 -> Product6/2
  Switch/1 -> Memory/1, Sum7/2
  Time 2/1 -> Sum9/2
  Switch1/1 -> Product6/1
  Clock1/1 -> Switch/2
  Memory/1 -> Switch/1
  Null 2/1 -> Switch1/1
  Divide3/1 -> Sum9/3, To Workspace6/1
  Clock2/1 -> Sum9/1
  In2/1 -> Sum7/1
  Vinj steady state/1 -> Sum8/1
  In3/1 -> Switch1/3, Divide3/2
  Sum9/1 -> Switch1/2
  Sum7/1 -> Sum8/2
  Product6/1 -> Out1/1
  Sum8/1 -> Divide3/1, To Workspace2/1

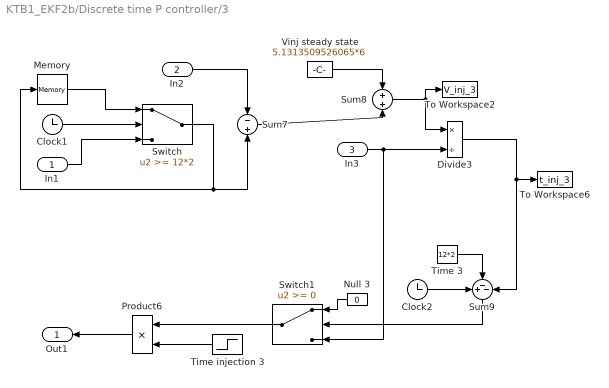
== system KTB1_EKF2b/Discrete time P controller/3 ==
  In1 : Inport
  In2 : Inport  Port=2
  In3 : Inport  Port=3
  Clock1 : Clock
  Clock2 : Clock
  Divide3 : Product  Inputs=*/
  Memory : Memory
  Null 3 : Constant  Value=0
  Product6 : Product
  Sum7 : Sum  Inputs=-+
  Sum8 : Sum
  Sum9 : Sum  Inputs=+--
  Switch : Switch  Threshold=12*2  SaturateOnIntegerOverflow=off  InputSameDT=off
  Switch1 : Switch  SaturateOnIntegerOverflow=off  InputSameDT=off
  Time 3 : Constant  Value=12*2
  Time injection 3 : Step  Time=12*2  SampleTime=0
  To Workspace2 : ToWorkspace  VariableName=V_inj_3  SaveFormat=Timeseries  SampleTime=-1
  To Workspace6 : ToWorkspace  VariableName=t_inj_3  SaveFormat=Timeseries  SampleTime=-1
  Vinj steady state : Constant  Value=5.1313509526065*6
  Out1 : Outport  VectorParamsAs1DForOutWhenUnconnected=off
  wires:
  In1/1 -> Switch/3
  Time injection 3/1 -> Product6/2
  Switch/1 -> Memory/1, Sum7/2
  Time 3/1 -> Sum9/2
  Switch1/1 -> Product6/1
  Clock1/1 -> Switch/2
  Memory/1 -> Switch/1
  Null 3/1 -> Switch1/1
  Divide3/1 -> Sum9/3, To Workspace6/1
  Clock2/1 -> Sum9/1
  In2/1 -> Sum7/1
  Vinj steady state/1 -> Sum8/1
  In3/1 -> Switch1/3, Divide3/2
  Sum9/1 -> Switch1/2
  Sum7/1 -> Sum8/2
  Product6/1 -> Out1/1
  Sum8/1 -> Divide3/1, To Workspace2/1

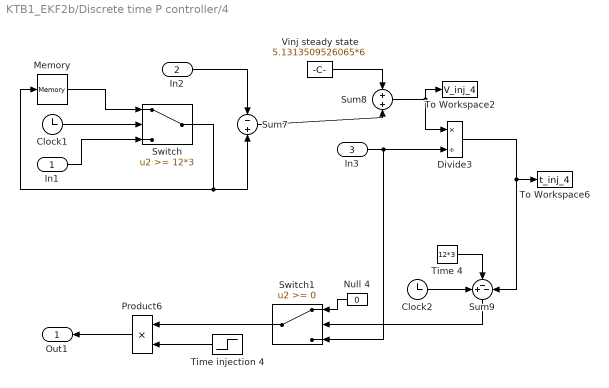
== system KTB1_EKF2b/Discrete time P controller/4 ==
  In1 : Inport
  In2 : Inport  Port=2
  In3 : Inport  Port=3
  Clock1 : Clock
  Clock2 : Clock
  Divide3 : Product  Inputs=*/
  Memory : Memory
  Null 4 : Constant  Value=0
  Product6 : Product
  Sum7 : Sum  Inputs=-+
  Sum8 : Sum
  Sum9 : Sum  Inputs=+--
  Switch : Switch  Threshold=12*3  SaturateOnIntegerOverflow=off  InputSameDT=off
  Switch1 : Switch  SaturateOnIntegerOverflow=off  InputSameDT=off
  Time 4 : Constant  Value=12*3
  Time injection 4 : Step  Time=12*3  SampleTime=0
  To Workspace2 : ToWorkspace  VariableName=V_inj_4  SaveFormat=Timeseries  SampleTime=-1
  To Workspace6 : ToWorkspace  VariableName=t_inj_4  SaveFormat=Timeseries  SampleTime=-1
  Vinj steady state : Constant  Value=5.1313509526065*6
  Out1 : Outport  VectorParamsAs1DForOutWhenUnconnected=off
  wires:
  In1/1 -> Switch/3
  Time injection 4/1 -> Product6/2
  Switch/1 -> Memory/1, Sum7/2
  Time 4/1 -> Sum9/2
  Switch1/1 -> Product6/1
  Clock1/1 -> Switch/2
  Memory/1 -> Switch/1
  Null 4/1 -> Switch1/1
  Divide3/1 -> Sum9/3, To Workspace6/1
  Clock2/1 -> Sum9/1
  In2/1 -> Sum7/1
  Vinj steady state/1 -> Sum8/1
  In3/1 -> Switch1/3, Divide3/2
  Sum9/1 -> Switch1/2
  Sum7/1 -> Sum8/2
  Product6/1 -> Out1/1
  Sum8/1 -> Divide3/1, To Workspace2/1

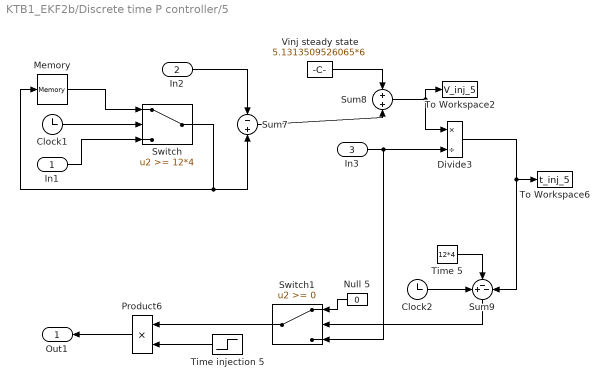
== system KTB1_EKF2b/Discrete time P controller/5 ==
  In1 : Inport
  In2 : Inport  Port=2
  In3 : Inport  Port=3
  Clock1 : Clock
  Clock2 : Clock
  Divide3 : Product  Inputs=*/
  Memory : Memory
  Null 5 : Constant  Value=0
  Product6 : Product
  Sum7 : Sum  Inputs=-+
  Sum8 : Sum
  Sum9 : Sum  Inputs=+--
  Switch : Switch  Threshold=12*4  SaturateOnIntegerOverflow=off  InputSameDT=off
  Switch1 : Switch  SaturateOnIntegerOverflow=off  InputSameDT=off
  Time 5 : Constant  Value=12*4
  Time injection 5 : Step  Time=12*4  SampleTime=0
  To Workspace2 : ToWorkspace  VariableName=V_inj_5  SaveFormat=Timeseries  SampleTime=-1
  To Workspace6 : ToWorkspace  VariableName=t_inj_5  SaveFormat=Timeseries  SampleTime=-1
  Vinj steady state : Constant  Value=5.1313509526065*6
  Out1 : Outport  VectorParamsAs1DForOutWhenUnconnected=off
  wires:
  In1/1 -> Switch/3
  Time injection 5/1 -> Product6/2
  Switch/1 -> Memory/1, Sum7/2
  Time 5/1 -> Sum9/2
  Switch1/1 -> Product6/1
  Clock1/1 -> Switch/2
  Memory/1 -> Switch/1
  Null 5/1 -> Switch1/1
  Divide3/1 -> Sum9/3, To Workspace6/1
  Clock2/1 -> Sum9/1
  In2/1 -> Sum7/1
  Vinj steady state/1 -> Sum8/1
  In3/1 -> Switch1/3, Divide3/2
  Sum9/1 -> Switch1/2
  Sum7/1 -> Sum8/2
  Product6/1 -> Out1/1
  Sum8/1 -> Divide3/1, To Workspace2/1

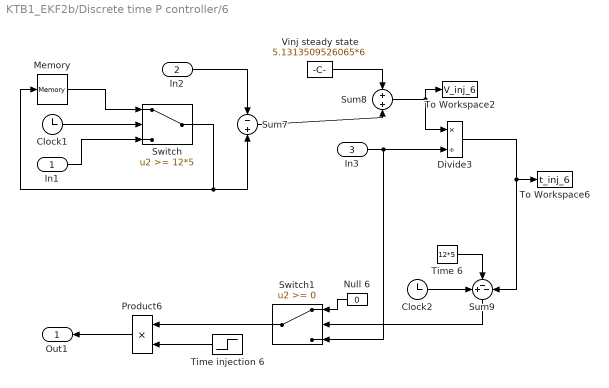
== system KTB1_EKF2b/Discrete time P controller/6 ==
  In1 : Inport
  In2 : Inport  Port=2
  In3 : Inport  Port=3
  Clock1 : Clock
  Clock2 : Clock
  Divide3 : Product  Inputs=*/
  Memory : Memory
  Null 6 : Constant  Value=0
  Product6 : Product
  Sum7 : Sum  Inputs=-+
  Sum8 : Sum
  Sum9 : Sum  Inputs=+--
  Switch : Switch  Threshold=12*5  SaturateOnIntegerOverflow=off  InputSameDT=off
  Switch1 : Switch  SaturateOnIntegerOverflow=off  InputSameDT=off
  Time 6 : Constant  Value=12*5
  Time injection 6 : Step  Time=12*5  SampleTime=0
  To Workspace2 : ToWorkspace  VariableName=V_inj_6  SaveFormat=Timeseries  SampleTime=-1
  To Workspace6 : ToWorkspace  VariableName=t_inj_6  SaveFormat=Timeseries  SampleTime=-1
  Vinj steady state : Constant  Value=5.1313509526065*6
  Out1 : Outport  VectorParamsAs1DForOutWhenUnconnected=off
  wires:
  In1/1 -> Switch/3
  Time injection 6/1 -> Product6/2
  Switch/1 -> Memory/1, Sum7/2
  Time 6/1 -> Sum9/2
  Switch1/1 -> Product6/1
  Clock1/1 -> Switch/2
  Memory/1 -> Switch/1
  Null 6/1 -> Switch1/1
  Divide3/1 -> Sum9/3, To Workspace6/1
  Clock2/1 -> Sum9/1
  In2/1 -> Sum7/1
  Vinj steady state/1 -> Sum8/1
  In3/1 -> Switch1/3, Divide3/2
  Sum9/1 -> Switch1/2
  Sum7/1 -> Sum8/2
  Product6/1 -> Out1/1
  Sum8/1 -> Divide3/1, To Workspace2/1

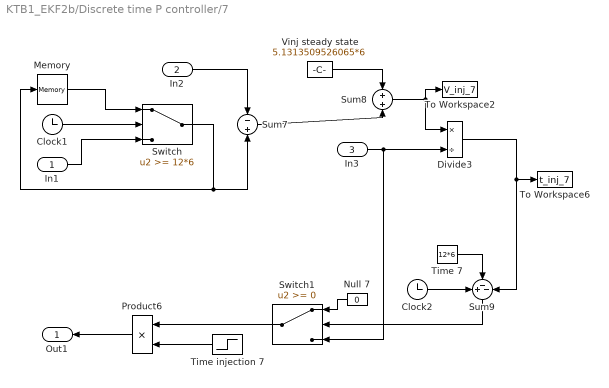
== system KTB1_EKF2b/Discrete time P controller/7 ==
  In1 : Inport
  In2 : Inport  Port=2
  In3 : Inport  Port=3
  Clock1 : Clock
  Clock2 : Clock
  Divide3 : Product  Inputs=*/
  Memory : Memory
  Null 7 : Constant  Value=0
  Product6 : Product
  Sum7 : Sum  Inputs=-+
  Sum8 : Sum
  Sum9 : Sum  Inputs=+--
  Switch : Switch  Threshold=12*6  SaturateOnIntegerOverflow=off  InputSameDT=off
  Switch1 : Switch  SaturateOnIntegerOverflow=off  InputSameDT=off
  Time 7 : Constant  Value=12*6
  Time injection 7 : Step  Time=12*6  SampleTime=0
  To Workspace2 : ToWorkspace  VariableName=V_inj_7  SaveFormat=Timeseries  SampleTime=-1
  To Workspace6 : ToWorkspace  VariableName=t_inj_7  SaveFormat=Timeseries  SampleTime=-1
  Vinj steady state : Constant  Value=5.1313509526065*6
  Out1 : Outport  VectorParamsAs1DForOutWhenUnconnected=off
  wires:
  In1/1 -> Switch/3
  Time injection 7/1 -> Product6/2
  Switch/1 -> Memory/1, Sum7/2
  Time 7/1 -> Sum9/2
  Switch1/1 -> Product6/1
  Clock1/1 -> Switch/2
  Memory/1 -> Switch/1
  Null 7/1 -> Switch1/1
  Divide3/1 -> Sum9/3, To Workspace6/1
  Clock2/1 -> Sum9/1
  In2/1 -> Sum7/1
  Vinj steady state/1 -> Sum8/1
  In3/1 -> Switch1/3, Divide3/2
  Sum9/1 -> Switch1/2
  Sum7/1 -> Sum8/2
  Product6/1 -> Out1/1
  Sum8/1 -> Divide3/1, To Workspace2/1

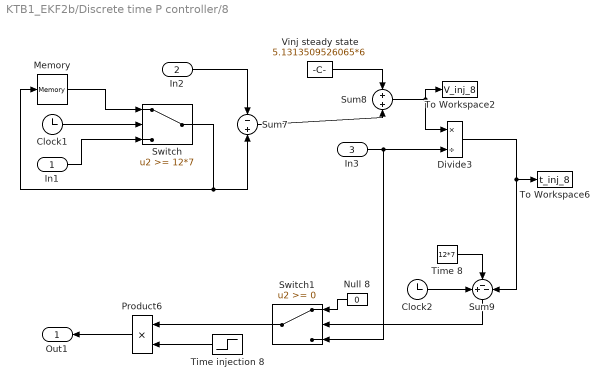
== system KTB1_EKF2b/Discrete time P controller/8 ==
  In1 : Inport
  In2 : Inport  Port=2
  In3 : Inport  Port=3
  Clock1 : Clock
  Clock2 : Clock
  Divide3 : Product  Inputs=*/
  Memory : Memory
  Null 8 : Constant  Value=0
  Product6 : Product
  Sum7 : Sum  Inputs=-+
  Sum8 : Sum
  Sum9 : Sum  Inputs=+--
  Switch : Switch  Threshold=12*7  SaturateOnIntegerOverflow=off  InputSameDT=off
  Switch1 : Switch  SaturateOnIntegerOverflow=off  InputSameDT=off
  Time 8 : Constant  Value=12*7
  Time injection 8 : Step  Time=12*7  SampleTime=0
  To Workspace2 : ToWorkspace  VariableName=V_inj_8  SaveFormat=Timeseries  SampleTime=-1
  To Workspace6 : ToWorkspace  VariableName=t_inj_8  SaveFormat=Timeseries  SampleTime=-1
  Vinj steady state : Constant  Value=5.1313509526065*6
  Out1 : Outport  VectorParamsAs1DForOutWhenUnconnected=off
  wires:
  In1/1 -> Switch/3
  Time injection 8/1 -> Product6/2
  Switch/1 -> Memory/1, Sum7/2
  Time 8/1 -> Sum9/2
  Switch1/1 -> Product6/1
  Clock1/1 -> Switch/2
  Memory/1 -> Switch/1
  Null 8/1 -> Switch1/1
  Divide3/1 -> Sum9/3, To Workspace6/1
  Clock2/1 -> Sum9/1
  In2/1 -> Sum7/1
  Vinj steady state/1 -> Sum8/1
  In3/1 -> Switch1/3, Divide3/2
  Sum9/1 -> Switch1/2
  Sum7/1 -> Sum8/2
  Product6/1 -> Out1/1
  Sum8/1 -> Divide3/1, To Workspace2/1

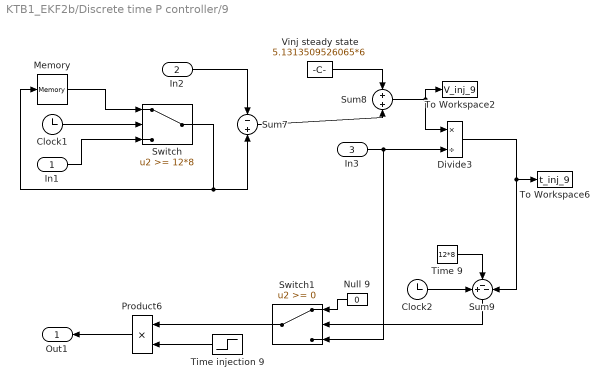
== system KTB1_EKF2b/Discrete time P controller/9 ==
  In1 : Inport
  In2 : Inport  Port=2
  In3 : Inport  Port=3
  Clock1 : Clock
  Clock2 : Clock
  Divide3 : Product  Inputs=*/
  Memory : Memory
  Null 9 : Constant  Value=0
  Product6 : Product
  Sum7 : Sum  Inputs=-+
  Sum8 : Sum
  Sum9 : Sum  Inputs=+--
  Switch : Switch  Threshold=12*8  SaturateOnIntegerOverflow=off  InputSameDT=off
  Switch1 : Switch  SaturateOnIntegerOverflow=off  InputSameDT=off
  Time 9 : Constant  Value=12*8
  Time injection 9 : Step  Time=12*8  SampleTime=0
  To Workspace2 : ToWorkspace  VariableName=V_inj_9  SaveFormat=Timeseries  SampleTime=-1
  To Workspace6 : ToWorkspace  VariableName=t_inj_9  SaveFormat=Timeseries  SampleTime=-1
  Vinj steady state : Constant  Value=5.1313509526065*6
  Out1 : Outport  VectorParamsAs1DForOutWhenUnconnected=off
  wires:
  In1/1 -> Switch/3
  Time injection 9/1 -> Product6/2
  Switch/1 -> Memory/1, Sum7/2
  Time 9/1 -> Sum9/2
  Switch1/1 -> Product6/1
  Clock1/1 -> Switch/2
  Memory/1 -> Switch/1
  Null 9/1 -> Switch1/1
  Divide3/1 -> Sum9/3, To Workspace6/1
  Clock2/1 -> Sum9/1
  In2/1 -> Sum7/1
  Vinj steady state/1 -> Sum8/1
  In3/1 -> Switch1/3, Divide3/2
  Sum9/1 -> Switch1/2
  Sum7/1 -> Sum8/2
  Product6/1 -> Out1/1
  Sum8/1 -> Divide3/1, To Workspace2/1

== matlab function KTB1_EKF2b/M-101 ==
  data: y output; u input
function y  = MX(u) 

% inputs
Q_R = u(1);
Q_M = u(2);
C_LAC_M = u(3);
C_N_M = u(4);
C_X_S = u(5);
C_LAC_S = u(6);
C_N_S = u(7);
C_MEV_S = u(8);

%C_LAC_M=10;
%C_N_M=2;

beta=1.9;

%remember C_LAC_R=C_LAC_S C_N_R=C_N_S

y=zeros(5,1);
y(1) = C_X_S*beta*Q_R/(Q_M+Q_R); %C_X_F
y(2) = (C_LAC_M*Q_M+C_LAC_S*Q_R)/(Q_M+Q_R); %C_LAC_F
y(3) = (C_N_M*Q_M+C_N_S*Q_R)/(Q_M+Q_R); %C_N_F
y(4) = C_MEV_S*Q_R/(Q_M+Q_R); %C_MEV_F
y(5) = (Q_M+Q_R); % Q_F

== matlab function KTB1_EKF2b/C-101 ==
  data: u input size=6; y output
 function y  = CF1(u)
% X=0.99; %separation factor
%Q4=QP1; volumetric capacity of the centrifuge

%inputs
C_X_T = u(1);
C_LAC_T = u(2);
C_N_T = u(3);
C_MEV_T = u(4);
Q_T = u(5);
X = u(6);

y=zeros(5,1);

y(1)=(1-X)*C_X_T;
y(2)=C_LAC_T;
y(3)=C_N_T;
y(4)=C_MEV_T;
y(5)= Q_T;

== matlab function KTB1_EKF2b/Purge ==
  data: u input size=7; y output
function y = PU(u)

% inputs
C_X_S = u(1);
C_LAC_S = u(2);
C_N_S = u(3);
C_MEV_S = u(4);
Q_M=u(5);
Q_C=u(6);
Q_P=u(7);

%F_purge=0.13;
%R=0.8;
% Q1=1.6; %l/h
%QC=1.8;
% F_purge*Q_C
%Q_P=Q_C-0.8*Q_1;

y=zeros(2,1);
y(1) = (Q_C-Q_P)/Q_M; % RR
y(2) = (Q_C-Q_P); % Q_R

== matlab function KTB1_EKF2b/C-102 ==
  data: u input size=6; y output
 function y  = CF2(u)
% X=0.99; %separation factor
%Q4=QP1; volumetric capacity of the centrifuge

%inputs
X = u(1); %separation factor
C_X_T = u(2);
C_LAC_T = u(3);
C_N_T = u(4);
C_MEV_T = u(5);
Q_T = u(6);


y=zeros(5,1);

y(1)=(1-X)*C_X_T;
y(2)=C_LAC_T;
y(3)=C_N_T;
y(4)=C_MEV_T;
y(5)= Q_T;

== matlab function KTB1_EKF2b/VSP-101 ==
  data: u input size=2; y output size=2
function y  = VSP(u)

%input
%time=u(1);
Q=u(1);
n=u(2);

dim=2;

y=zeros(dim,1);

% output

y(1)=Q;
y(2)=(-0.085*Q^2 - 0.0000329*Q*n + 0.0000155555555555556*n^2)/10.2024665317458;

% -0.085x^(2)-0.0000329*2900x+0.0000155555555555556*2900

%10.199773339984

end

== matlab function KTB1_EKF2b/NF-101 ==
  data: u input size=5; y output size=9
function y  = NF(u)
%% parameters for nanofiltration 
% a DOW NF90 nanofiltration membrane has been chosen. This type of membrane
% has been used in pharmaceutical applications for API filtrations (title
% reference: Removal of antibiotics from a model wastewater by RO/NF membranes)
%A=0.398443840087261; %membrane surface area [m^2] 
A=0.3984033;
Jw=57.90; %permeate flowrate at 8 bar pressure [l/m^2/h]
Res=Jw/8; %[l/m^2/h/bar]
% [LAC N MEV-H]


%input
C_LAC_4=u(1);
C_N_4=u(2);
C_MEV_4=u(3);
Q_IN=u(4);
P=u(5);


tlim=1; %h
dim=9;

y=zeros(dim,1);

%rejection factors based on molecular weights of similar compounds
if P<=8
    Rej=[0.9; 0.79; 0.00002*P^4 - 0.0018*P^3 + 0.0145*P^2 + 0.0849*P + 0.22248];
else
    Rej=[0.9; 0.79; 0.00002*8^4 - 0.0018*8^3 + 0.0145*8^2 + 0.0849*8 + 0.22248];
end
%Rej=[0.9; 0.79; 0.99];
% y=zeros(4,1);
% tlim=500;

%% output
%y=[Q_P2,Q_R,C_LAC_R,C_N_R,C_MEV_R,C_LAC_P2,C_N_P2,C_MEV_P2]
% if time>=0 && time<tlim
    y(1)=A*Res*P;%permeate volumetric flowrate [l/h];(ref: Continuous purification of
    %active pharmaceutical ingredients using multistage organic solvent nanofiltration membrane cascade)
    y(2)=Q_IN-y(1); %balance on centrifugation+filtration
    y(3)=(Q_IN*C_LAC_4)/(y(2)+y(1)*(1-Rej(1)));%species balance--retentate stream
    y(4)=(Q_IN*C_N_4)/(y(2)+y(1)*(1-Rej(2)));%species balance--retentate stream
    y(5)=(Q_IN*C_MEV_4)/(y(2)+y(1)*(1-Rej(3)));%species balance--retentate stream
    y(6)=y(3)*(1-Rej(1));%LAC
    y(7)=y(4)*(1-Rej(2));%N
    y(8)=y(5)*(1-Rej(3));%MEV
    y(9)=Rej(3);
%else
%    for i=1:dim
%        y(i)=0;
%    end
%end
end

== matlab function KTB1_EKF2b/HC-101 ==
  data: u input; y output
function y  = HC(u)

%inputs
Q_S=u(1);
Q_C=u(2);
C_X_S=u(3);
C_LAC_S=u(4);
C_N_S=u(5);
C_MEV_S=u(6);
% Q_R=u(7); % Serve soltanto per Fpurge, eliminabile

%parameters
%R=0.8;
beta=1.6;
%F_purge=0.13;

y=zeros(5,1);

y(1) = (C_X_S*Q_S-beta*C_X_S*Q_C)/(Q_S-Q_C); % C_X
y(2) = C_LAC_S;
y(3) = C_N_S;
y(4) = C_MEV_S;
%y(5) = 1-Q_R/Q_C;
y(5) = Q_S-Q_C;

== matlab function KTB1_EKF2b/Controller settings ==
  data: u input size=1; y output size=4
function y  = CN(u)

%inputs
err=u(1);

y=zeros(4,1);
y(1) = -2411.68044009728/310 -30*err; % P
y(2) = y(1)/599.84*1.7; % I
y(3) = -721.322122263916; % D
y(4) = 0.41482994666475; % N
